simulink library "stabilizerController_ul"  (R2018a)
settings: Solver=VariableStepAuto  StartTime=0.0  StopTime=10.0  RelTol=1e-3
undefined symbols (not defined in the file): iterationPhase_enum, plant
libraries: simulink x2
settings Model: Creator=mitch  LastModifiedBy=mitch

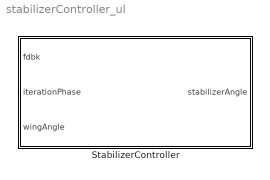
== system stabilizerController_ul ==
  StabilizerController : Subsystem

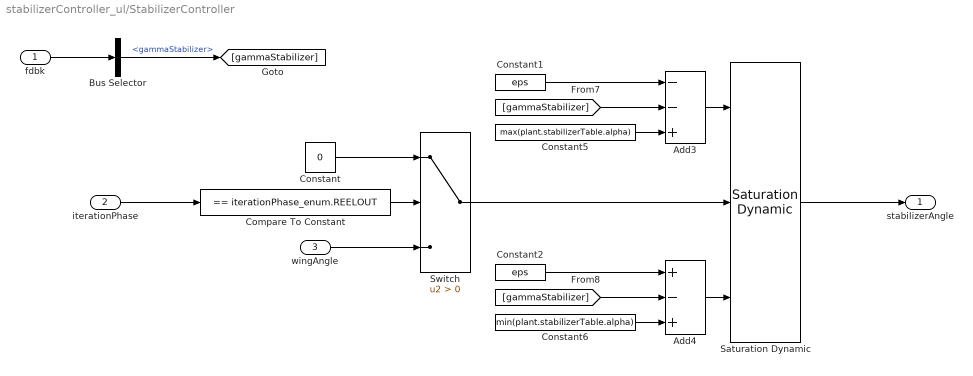
== system stabilizerController_ul/StabilizerController ==
  fdbk : Inport  OutDataTypeStr=Bus: busPlantFeedback
  iterationPhase : Inport  Port=2
  wingAngle : Inport  Port=3
  Add3 : Sum  Inputs=--+
  Add4 : Sum  Inputs=+-+
  Bus Selector : BusSelector  OutputSignals=gammaStabilizer
  Compare To Constant : simulink/Logic and Bit Operations/Compare To Constant  relop===  const=iterationPhase_enum.REELOUT  OutDataTypeStr=boolean
  Constant : Constant  Value=0
  Constant1 : Constant  Value=eps
  Constant2 : Constant  Value=eps
  Constant5 : Constant  Value=max(plant.stabilizerTable.alpha)
  Constant6 : Constant  Value=min(plant.stabilizerTable.alpha)
  Saturation Dynamic : simulink/Discontinuities/Saturation Dynamic  OutMin=[]  OutMax=[]  OutDataTypeStr=Inherit: Same as second input  OutDataType=fixdt(1, 16)  OutScaling=2^-10  DoSatur=off
  Switch : Switch  Criteria=u2 > Threshold
  stabilizerAngle : Outport
  wires:
  Add3/1 -> Saturation Dynamic/1
  [gammaStabilizer] -> Add4/2
  Constant2/1 -> Add4/1
  fdbk/1 -> Bus Selector/1
  [gammaStabilizer] -> Add3/2
  Saturation Dynamic/1 -> stabilizerAngle/1
  Bus Selector/1 -> [gammaStabilizer]  "<gammaStabilizer>"
  Constant1/1 -> Add3/1
  iterationPhase/1 -> Compare To Constant/1
  Switch/1 -> Saturation Dynamic/2
  Add4/1 -> Saturation Dynamic/3
  Constant6/1 -> Add4/3
  Constant5/1 -> Add3/3
  Compare To Constant/1 -> Switch/2
  Constant/1 -> Switch/1
  wingAngle/1 -> Switch/3
